simulink model "VL53L8A1_Full"  (R2024b)
settings: Solver=FixedStepDiscrete  StartTime=0.0  StopTime=inf  RelTol=1e-3  EnableMultiTasking=on
PreLoadFcn:
  | addpath(genpath(pwd))
InitFcn:
  | addpath(genpath(pwd));
  | auto_program("VL53L8A1_Full");
  | STLINK_COMPORT = auto_COMPORT()
  | 
  | dialogPrms = get_param(gcs+"/VL53L8A1", 'DialogParameters');
  | dialogPrmNames = fieldnames(dialogPrms);
  | odr4 = get_param(gcs+"/VL53L8A1", dialogPrmNames{1});
  | odr4 = eval(odr4);
  | 
  | STM32_ODR = odr4
  | clearvars -except STLINK_COMPORT STLINK_DRIVE STM32_ODR
libraries: instrumentseriallib x3, etargetslib x3
settings Model: SimulationMode=accelerator  PacingRate=0.100000  ExtModeTrigDuration=10  Creator=JesseJabezArendse  LastModifiedBy=JesseJabezArendse
settings OptimizationCC: ReuseModelBlockBuffer=off  PassReuseOutputArgsAs=Individual arguments  ZeroExternalMemoryAtStartup=off  ZeroInternalMemoryAtStartup=off  MaxStackSize=64  OptimizationLevel=level1  OptimizationCustomize=off  EfficientTunableParamExpr=on
settings DebuggingCC: ParameterPrecisionLossMsg=none  ParameterTunabilityLossMsg=error
settings HardwareCC: ProdBitPerPointer=32  ProdBitPerSizeT=32  ProdBitPerPtrDiffT=32  ProdLargestAtomicInteger=Long  ProdLargestAtomicFloat=Double  ProdWordSize=32  ProdLongLongMode=on  ProdHWDeviceType=ARM Compatible->ARM Cortex
settings ModelReferenceCC: EnableParallelModelReferenceBuilds=on
settings SFSimCC: SimCustomHeaderCode="#include \"Core\\Inc\\main.h\""  SimParseCustomCode=off  MATLABDynamicMemAlloc=off  SimHardwareAcceleration=native
settings SFSimCC: SimUserSources=|
  | Core\Src\main.c
  | Core\Src\IKS02A1_Simulink.c
settings SFSimCC: SimUserIncludeDirs=|
  | Core\Inc\
  | Core\Src\
settings RTWCC: Description=Embedded Coder  SystemTargetFile=ert.tlc  TemplateMakefile=ert_default_tmf  RTWUseSimCustomCode=on  CustomHeaderCode="#include \"Core\\Inc\\main.h\""  Toolchain=GNU Tools for ARM Embedded Processors  BuildConfiguration=Specify  GPUComputeCapability=3.5
settings RTWCC: CustomInclude=|
  | Core\Inc\
  | Core\Src\
settings RTWCC: CustomSource=|
  | Core\Src\main.c
  | Core\Src\IKS02A1_Simulink.c
settings CodeAppCC: ForceParamTrailComments=on  IgnoreCustomStorageClasses=off  OperatorAnnotations=on  SimulinkDataObjDesc=on  SFDataObjDesc=on  InsertBlockDesc=on
settings ERTTargetCC: CodeReplacementLibrary=ARM Cortex-M  SupportContinuousTime=on  ExtModeTransport=3  ExtModeStaticAlloc=on  ExtModeStaticAllocSize=2000  ExtModeMexFile=ext_xcp  ExtModeIntrfLevel=Level2 - Open  InlinedParameterPlacement=Hierarchical  ERTCustomFileTemplate=example_file_process.tlc  DynamicArrayContainerType=coder::array

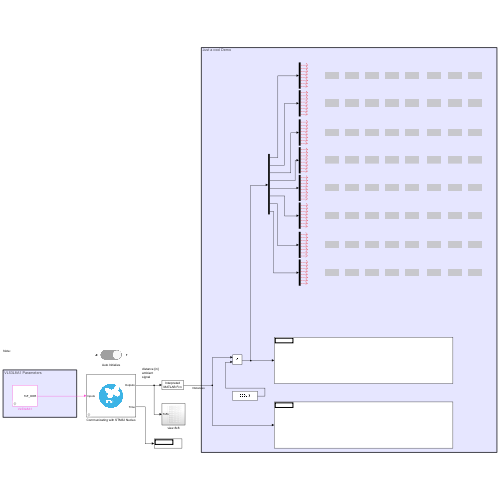
[thumbnail: Simulink's stored preview of the top-level diagram]
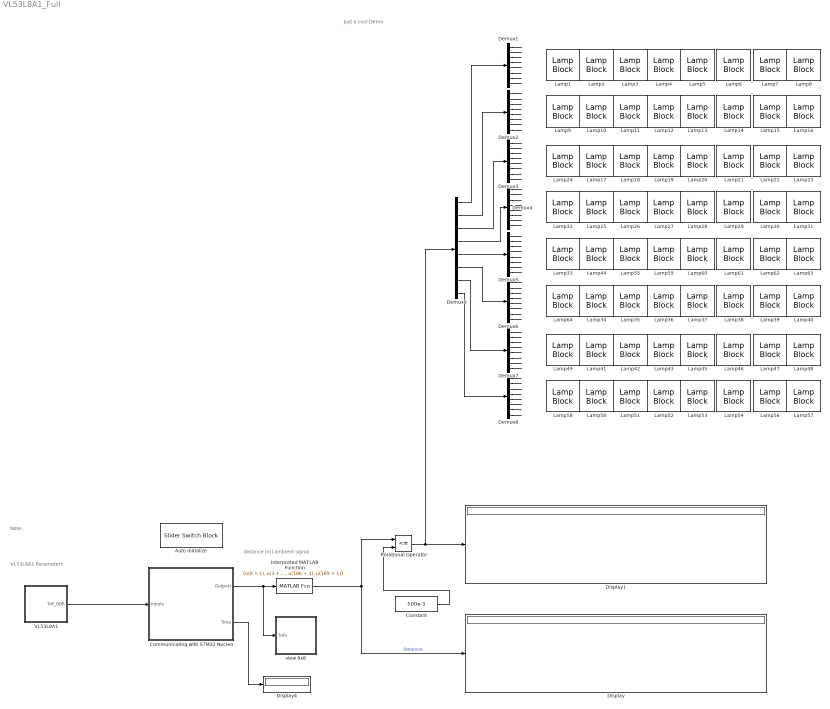
== system VL53L8A1_Full ==
  note: Just a cool Demo
  note: distance [m]
      | ambient
      | signal
  note: Note:
  note: VL53L8A1 Parameters
  Auto Initialize : SliderSwitchBlock  LabelPosition=Hide
      settings: Values={{'Off', 'On'}, [0 1]}
  Communicating with STM32 Nucleo : Subsystem  mask{Auto_Initialize=1}
      mask prompts: Auto_Initialize "Automate Initialization?"
      mask TypeOptions Auto_Initialize: 1 | 0
      mask DialogControl Control1 Prompt: Block for communication between host machine and STM32 Nucleo F411RE
      mask Display: image('stm32_icon.png', [0,0,0,0,80,80]);
  Constant : Constant  Value=500e-3
  Demux0 : Demux  Outputs=[8 8 8 8 8 8 8 8]
  Demux{1..8} (8 alike) : Demux  Outputs=[1 1 1 1 1 1 1 1]
  Display : Display
  Display1 : Display
  Display4 : Display
  Interpreted MATLAB Function : MATLABFcn  MATLABFcn=|
      | [u(0 + 1),
      | u(3 + 1),
      | u(6 + 1),
      | u(9 + 1),
      | u(12 + 1),
      | u(15 + 1),
      | u(18 + 1),
      | u(21 + 1),
      | u(24 + 1),
      | u(27 + 1),
      | u(30 + 1),
      | u(33 + 1),
      | u(36 + 1),
      | u(39 + 1),
      | u(42 + 1),
      | u(45 + 1),
      | u(48 + 1),
      | u(51 + 1),
      | u(54 + 1),
      | u(57 + 1),
      | u(60 + 1),
      | u(63 + 1),
      | u(66 + 1),
      | u(69 + 1),
      | u(72 + 1),
      | u(75 + 1),
      | u(78 + 1),
      | u(81 + 1),
      | u(84 + 1),
      | u(87 + 1),
      | u(90 + 1),
      | u(93 + 1),
      | u(96 + 1),
      | u(99 + 1),
      | u(102 + 1),
      | u(105 + 1),
      | u(108 + 1),
      | u(111 + 1),
      | u(114 + 1),
      | u(117 + 1),
      | u(120 + 1),
      | u(123 + 1),
      | u(126 + 1),
      | u(129 + 1),
      | u(132 + 1),
      | u(135 + 1),
      | u(138 + 1),
      | u(141 + 1),
      | u(144 + 1),
      | u(147 + 1),
      | u(150 + 1),
      | u(153 + 1),
      | u(156 + 1),
      | u(159 + 1),
      | u(162 + 1),
      | u(165 + 1),
      | u(168 + 1),
      | u(171 + 1),
      | u(174 + 1),
      | u(177 + 1),
      | u(180 + 1),
      | u(183 + 1),
      | u(186 + 1),
      | u(189 + 1)]
  Lamp{1..64} (64 alike) : LampBlock  LabelPosition=Hide  Icon=Rectangle
  Relational Operator : RelationalOperator  Operator=<=  OutDataTypeStr=boolean  RndMeth=Simplest  InputSameDT=off
  VL53L8A1 : Subsystem  mask{ODR_TOF=20}
      mask prompts: ODR_TOF "Output Data Rate (Hz)"
      mask DialogControl DescGroupVar Prompt: Time of Flight Sensor 8x8
  view 8x8 : Subsystem
  wires:
  Interpreted MATLAB Function/1 -> Relational Operator/1, Display/1  "Distances"
  Constant/1 -> Relational Operator/2
  Demux1/1 -> ?
  Demux1/2 -> ?
  Demux1/3 -> ?
  Demux1/4 -> ?
  Demux1/5 -> ?
  Demux1/6 -> ?
  Demux1/7 -> ?
  Demux1/8 -> ?
  Relational Operator/1 -> Display1/1, Demux0/1
  Demux0/1 -> Demux1/1
  Demux2/8 -> ?
  Demux2/7 -> ?
  Demux2/6 -> ?
  Demux2/5 -> ?
  Demux2/4 -> ?
  Demux2/3 -> ?
  Demux2/2 -> ?
  Demux2/1 -> ?
  Demux0/2 -> Demux2/1
  Demux3/1 -> ?
  Demux3/3 -> ?
  Demux3/6 -> ?
  Demux3/2 -> ?
  Demux3/4 -> ?
  Demux3/5 -> ?
  Demux3/8 -> ?
  Demux0/3 -> Demux3/1
  Demux3/7 -> ?
  Demux4/2 -> ?
  Demux4/6 -> ?
  Demux4/1 -> ?
  Demux4/8 -> ?
  Demux4/5 -> ?
  Demux4/3 -> ?
  Demux4/7 -> ?
  Demux4/4 -> ?
  Demux0/4 -> Demux4/1
  Demux6/1 -> ?
  Demux6/2 -> ?
  Demux6/7 -> ?
  Demux6/4 -> ?
  Demux6/8 -> ?
  Demux5/3 -> ?
  Demux5/5 -> ?
  Demux6/6 -> ?
  Demux5/6 -> ?
  Demux7/2 -> ?
  Demux7/6 -> ?
  Demux6/3 -> ?
  Demux7/1 -> ?
  Demux5/7 -> ?
  Demux6/5 -> ?
  Demux5/8 -> ?
  Demux7/5 -> ?
  Demux7/8 -> ?
  Demux8/4 -> ?
  Demux8/1 -> ?
  Demux8/8 -> ?
  Demux7/7 -> ?
  Demux7/4 -> ?
  Demux8/3 -> ?
  Demux5/4 -> ?
  Demux8/7 -> ?
  Demux8/6 -> ?
  Demux7/3 -> ?
  Demux8/5 -> ?
  Demux8/2 -> ?
  Demux5/1 -> ?
  Demux5/2 -> ?
  Demux0/5 -> Demux5/1
  Demux0/6 -> Demux6/1
  Demux0/7 -> Demux7/1
  Demux0/8 -> Demux8/1
  Communicating with STM32 Nucleo/2(Time) -> Display4/1
  Communicating with STM32 Nucleo/1(Outputs) -> view 8x8/1(ToFs), Interpreted MATLAB Function/1
  VL53L8A1/1(ToF_ODR) -> Communicating with STM32 Nucleo/1(Inputs)

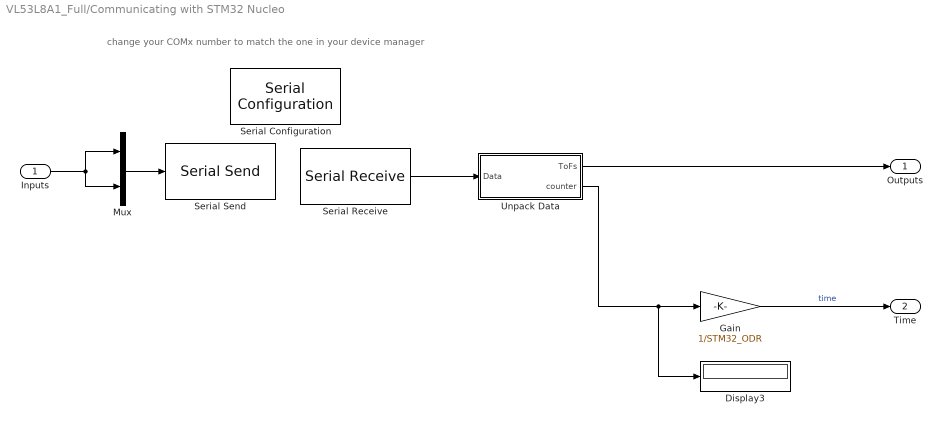
== system VL53L8A1_Full/Communicating with STM32 Nucleo ==
  note: change your COMx number to match the one in your device manager
  Inputs : Inport
  Display3 : Display
  Gain : Gain  Gain=1/STM32_ODR
  Mux : Mux  Inputs=2
  Serial Configuration : instrumentseriallib/Serial Configuration  Priority=-200000  PortSel=STLINK_COMPORT  Port=STLINK_COMPORT  ComPort=STLINK_COMPORT  BaudRate=1843200  DataBits=8  Parity=even  StopBits=2  ByteOrder=little-endian  FlowControl=none  Timeout=5  SimulateUsing=Interpreted execution  BlockInModel=on  aMode=1
      settings: LibrarySourceBlock=embeddedtargetslib/Host Communication/Serial Configuration
  Serial Receive : instrumentseriallib/Serial Receive  Priority=1  PortSel=STLINK_COMPORT  Port=STLINK_COMPORT  ComPort=STLINK_COMPORT  DataType=single  SaveDataType=uint8  ToggleHeader=on  Header='J_A'  ToggleDataSize=on  DataSize=[1 8*8*3+1]  ToggleTerminator=on  Terminator=Custom terminator  CustomTerminator='A_J'  InputFormat=Column major  EnableBlockingMode=on  ActionDataUnavailable=Output last received value  ActionWhenDataUnavailable=Output last received value  CustomValue=0  SampleTime=1/STM32_ODR  SimulateUsing=Interpreted execution  BlockInModel=on  aMode=1
      settings: LibrarySourceBlock=embeddedtargetslib/Host Communication/Serial Receive
  Serial Send : instrumentseriallib/Serial Send  Priority=1  PortSel=STLINK_COMPORT  Port=STLINK_COMPORT  ComPort=STLINK_COMPORT  Header='J_A'  Terminator=Custom terminator  CustomTerminator='A_J'  EnableBlockingMode=off  SimulateUsing=Interpreted execution  BlockInModel=on  aMode=1
      settings: LibrarySourceBlock=embeddedtargetslib/Host Communication/Serial Send
  Unpack Data : Subsystem
  Outputs : Outport
  Time : Outport  Port=2
  wires:
  Serial Receive/1 -> Unpack Data/1(Data)
  Gain/1 -> Time/1  "time"
  Inputs/1 -> Mux/1, Mux/2
  Unpack Data/1(ToFs) -> Outputs/1
  Unpack Data/2(counter) -> Gain/1, Display3/1
  Mux/1 -> Serial Send/1

== system VL53L8A1_Full/VL53L8A1 ==
  Byte Pack3 : etargetslib/Byte Pack  datatypes={'single'}  byteAlign=1
  Cast5 : DataTypeConversion  OutDataTypeStr=single  SaturateOnIntegerOverflow=off  RndMeth=Floor
  Constant1 : Constant  Value=ODR_TOF
  Display1 : Display
  ToF_ODR : Outport
  wires:
  Constant1/1 -> Cast5/1, Display1/1
  Cast5/1 -> Byte Pack3/1
  Byte Pack3/1 -> ToF_ODR/1

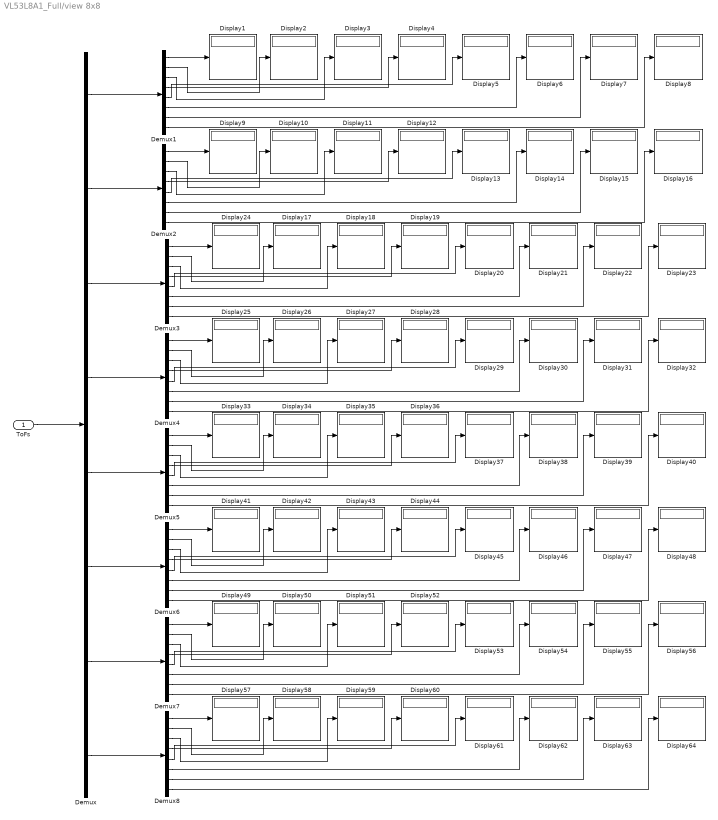
== system VL53L8A1_Full/view 8x8 ==
  ToFs : Inport
  Demux : Demux  Outputs=[3*8 3*8 3*8 3*8 3*8 3*8 3*8 3*8]
  Demux{1..8} (8 alike) : Demux  Outputs=[3 3 3 3 3 3 3 3]
  Display{1..64} (64 alike) : Display
  wires:
  Demux5/7 -> Display39/1
  Demux4/2 -> Display26/1
  Demux3/3 -> Display18/1
  Demux8/6 -> Display62/1
  Demux3/2 -> Display17/1
  Demux2/2 -> Display10/1
  Demux/5 -> Demux5/1
  Demux1/5 -> Display5/1
  Demux4/4 -> Display28/1
  Demux4/7 -> Display31/1
  Demux4/6 -> Display30/1
  Demux7/7 -> Display55/1
  Demux3/4 -> Display19/1
  Demux/8 -> Demux8/1
  Demux4/8 -> Display32/1
  Demux/4 -> Demux4/1
  Demux8/8 -> Display64/1
  Demux8/3 -> Display59/1
  Demux3/8 -> Display23/1
  Demux4/3 -> Display27/1
  Demux6/4 -> Display44/1
  Demux5/1 -> Display33/1
  Demux1/3 -> Display3/1
  Demux3/7 -> Display22/1
  Demux3/6 -> Display21/1
  Demux1/2 -> Display2/1
  Demux3/5 -> Display20/1
  Demux8/2 -> Display58/1
  Demux/1 -> Demux1/1
  Demux3/1 -> Display24/1
  Demux/2 -> Demux2/1
  Demux7/3 -> Display51/1
  Demux2/5 -> Display13/1
  Demux4/1 -> Display25/1
  Demux1/6 -> Display6/1
  Demux1/8 -> Display8/1
  Demux2/3 -> Display11/1
  Demux5/4 -> Display36/1
  Demux7/6 -> Display54/1
  Demux4/5 -> Display29/1
  Demux/6 -> Demux6/1
  Demux/3 -> Demux3/1
  Demux7/5 -> Display53/1
  Demux5/8 -> Display40/1
  Demux8/7 -> Display63/1
  Demux6/7 -> Display47/1
  Demux5/2 -> Display34/1
  Demux1/7 -> Display7/1
  Demux8/4 -> Display60/1
  Demux6/1 -> Display41/1
  Demux5/5 -> Display37/1
  Demux6/3 -> Display43/1
  Demux6/6 -> Display46/1
  Demux6/2 -> Display42/1
  Demux6/5 -> Display45/1
  Demux1/1 -> Display1/1
  Demux6/8 -> Display48/1
  Demux1/4 -> Display4/1
  Demux8/1 -> Display57/1
  Demux5/6 -> Display38/1
  Demux8/5 -> Display61/1
  Demux5/3 -> Display35/1
  Demux2/8 -> Display16/1
  Demux7/4 -> Display52/1
  Demux7/8 -> Display56/1
  Demux7/1 -> Display49/1
  Demux7/2 -> Display50/1
  Demux2/7 -> Display15/1
  Demux2/6 -> Display14/1
  Demux2/1 -> Display9/1
  Demux2/4 -> Display12/1
  Demux/7 -> Demux7/1
  ToFs/1 -> Demux/1

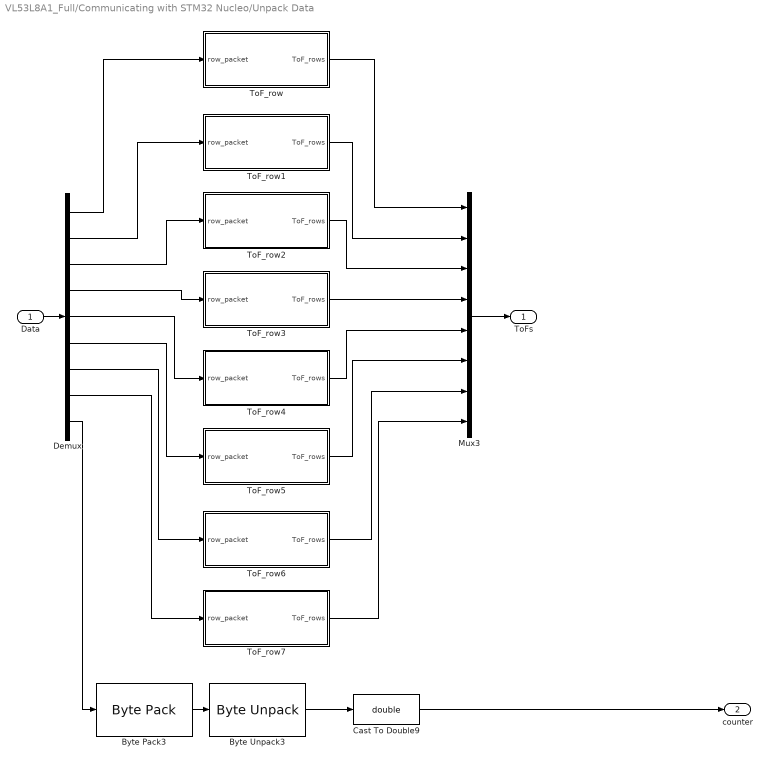
== system VL53L8A1_Full/Communicating with STM32 Nucleo/Unpack Data ==
  Data : Inport
  Byte Pack3 : etargetslib/Byte Pack  datatypes={'single'}  byteAlign=1
  Byte Unpack3 : etargetslib/Byte Unpack  dimensions={[1]}  datatypes={'uint32'}  byteAlign=1
      settings: LibrarySourceBlock=embeddedtargetslib/Host Communication/Byte Unpack
  Cast To Double9 : DataTypeConversion  OutDataTypeStr=double  SaturateOnIntegerOverflow=off  RndMeth=Floor
  Demux : Demux  Outputs=[3*8 3*8 3*8 3*8 3*8 3*8 3*8 3*8 1]
  Mux3 : Mux  Inputs=[3*8 3*8 3*8 3*8 3*8 3*8 3*8 3*8]
  ToF_row : Subsystem
  ToF_row1 : Subsystem
  ToF_row2 : Subsystem
  ToF_row3 : Subsystem
  ToF_row4 : Subsystem
  ToF_row5 : Subsystem
  ToF_row6 : Subsystem
  ToF_row7 : Subsystem
  ToFs : Outport
  counter : Outport  Port=2
  wires:
  Data/1 -> Demux/1
  Demux/7 -> ToF_row6/1(row_packet)
  Demux/6 -> ToF_row5/1(row_packet)
  Demux/5 -> ToF_row4/1(row_packet)
  Mux3/1 -> ToFs/1
  Demux/4 -> ToF_row3/1(row_packet)
  Demux/3 -> ToF_row2/1(row_packet)
  Demux/2 -> ToF_row1/1(row_packet)
  Demux/1 -> ToF_row/1(row_packet)
  Demux/8 -> ToF_row7/1(row_packet)
  ToF_row/1(ToF_rows) -> Mux3/1
  ToF_row1/1(ToF_rows) -> Mux3/2
  ToF_row2/1(ToF_rows) -> Mux3/3
  ToF_row3/1(ToF_rows) -> Mux3/4
  ToF_row4/1(ToF_rows) -> Mux3/5
  ToF_row5/1(ToF_rows) -> Mux3/6
  ToF_row6/1(ToF_rows) -> Mux3/7
  ToF_row7/1(ToF_rows) -> Mux3/8
  Demux/9 -> Byte Pack3/1
  Byte Unpack3/1 -> Cast To Double9/1
  Cast To Double9/1 -> counter/1
  Byte Pack3/1 -> Byte Unpack3/1

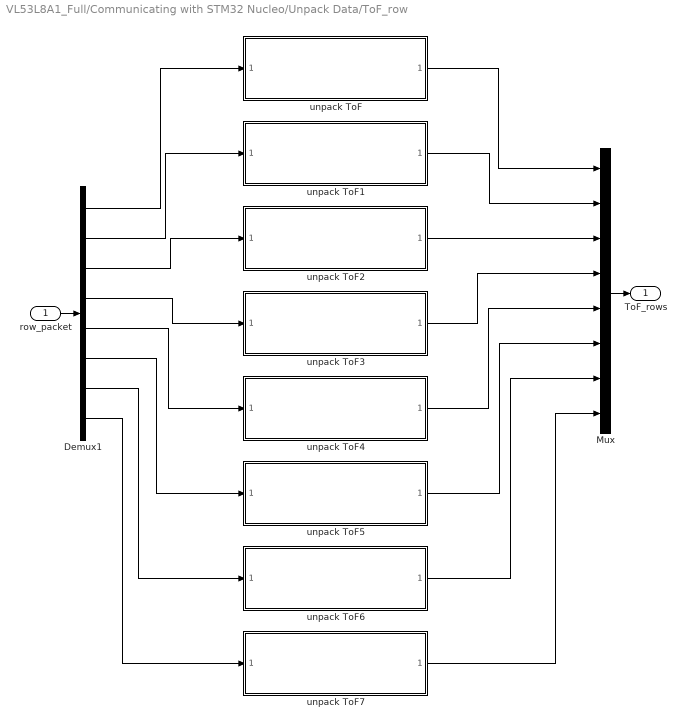
== system VL53L8A1_Full/Communicating with STM32 Nucleo/Unpack Data/ToF_row ==
  row_packet : Inport
  Demux1 : Demux  Outputs=[3 3 3 3 3 3 3 3]
  Mux : Mux  Inputs=[3 3 3 3 3 3 3 3]
  unpack ToF{,1..7} (8 alike) : Subsystem  ReferencedSubsystem=unpack_ToF
  ToF_rows : Outport
  wires:
  Demux1/7 -> unpack ToF6/1
  unpack ToF5/1 -> Mux/6
  unpack ToF3/1 -> Mux/4
  Demux1/1 -> unpack ToF/1
  Demux1/8 -> unpack ToF7/1
  Demux1/3 -> unpack ToF2/1
  Demux1/5 -> unpack ToF4/1
  Demux1/2 -> unpack ToF1/1
  unpack ToF1/1 -> Mux/2
  Demux1/4 -> unpack ToF3/1
  unpack ToF4/1 -> Mux/5
  unpack ToF7/1 -> Mux/8
  Mux/1 -> ToF_rows/1
  Demux1/6 -> unpack ToF5/1
  unpack ToF6/1 -> Mux/7
  unpack ToF/1 -> Mux/1
  unpack ToF2/1 -> Mux/3
  row_packet/1 -> Demux1/1

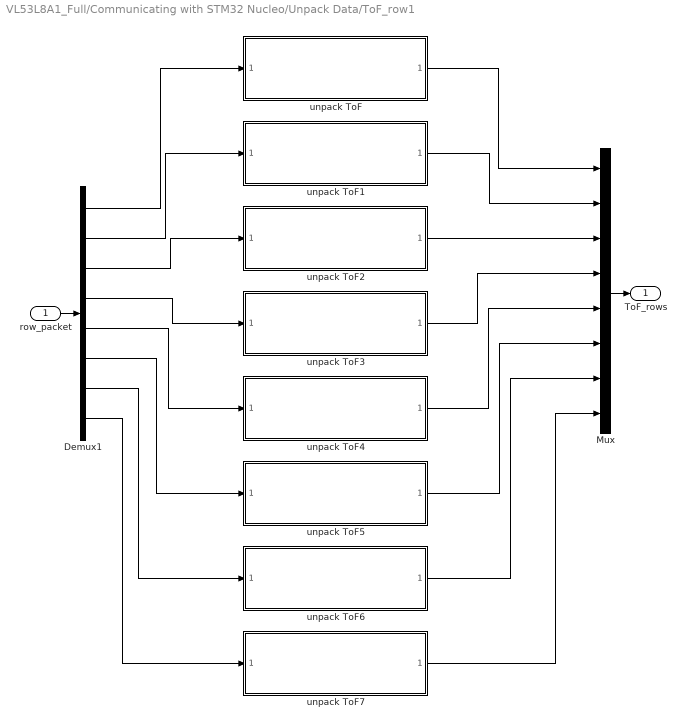
== system VL53L8A1_Full/Communicating with STM32 Nucleo/Unpack Data/ToF_row1 ==
  row_packet : Inport
  Demux1 : Demux  Outputs=[3 3 3 3 3 3 3 3]
  Mux : Mux  Inputs=[3 3 3 3 3 3 3 3]
  unpack ToF{,1..7} (8 alike) : Subsystem  ReferencedSubsystem=unpack_ToF
  ToF_rows : Outport
  wires:
  row_packet/1 -> Demux1/1
  unpack ToF2/1 -> Mux/3
  unpack ToF/1 -> Mux/1
  unpack ToF6/1 -> Mux/7
  Demux1/6 -> unpack ToF5/1
  Mux/1 -> ToF_rows/1
  unpack ToF7/1 -> Mux/8
  unpack ToF4/1 -> Mux/5
  Demux1/4 -> unpack ToF3/1
  unpack ToF1/1 -> Mux/2
  Demux1/2 -> unpack ToF1/1
  Demux1/5 -> unpack ToF4/1
  Demux1/3 -> unpack ToF2/1
  Demux1/8 -> unpack ToF7/1
  Demux1/1 -> unpack ToF/1
  unpack ToF3/1 -> Mux/4
  unpack ToF5/1 -> Mux/6
  Demux1/7 -> unpack ToF6/1

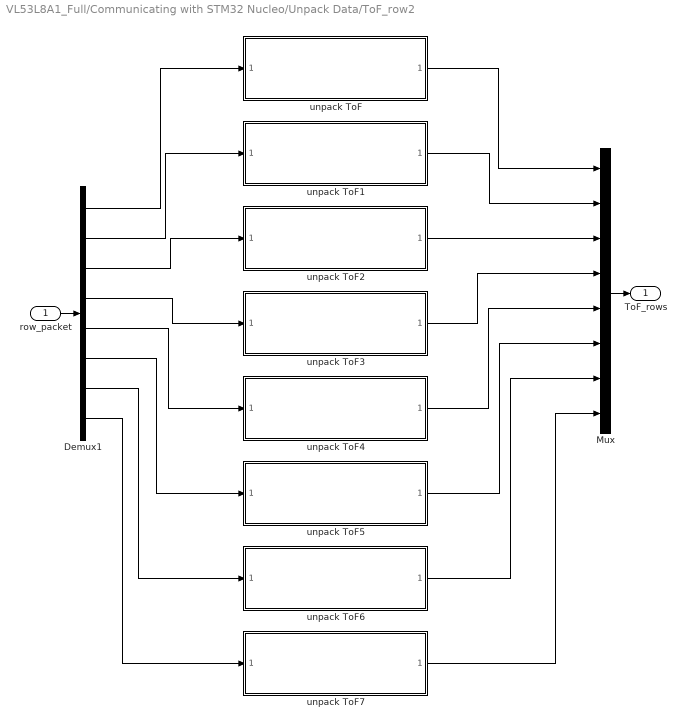
== system VL53L8A1_Full/Communicating with STM32 Nucleo/Unpack Data/ToF_row2 ==
  row_packet : Inport
  Demux1 : Demux  Outputs=[3 3 3 3 3 3 3 3]
  Mux : Mux  Inputs=[3 3 3 3 3 3 3 3]
  unpack ToF{,1..7} (8 alike) : Subsystem  ReferencedSubsystem=unpack_ToF
  ToF_rows : Outport
  wires:
  Demux1/7 -> unpack ToF6/1
  unpack ToF5/1 -> Mux/6
  unpack ToF3/1 -> Mux/4
  Demux1/1 -> unpack ToF/1
  Demux1/8 -> unpack ToF7/1
  Demux1/3 -> unpack ToF2/1
  Demux1/5 -> unpack ToF4/1
  Demux1/2 -> unpack ToF1/1
  unpack ToF1/1 -> Mux/2
  Demux1/4 -> unpack ToF3/1
  unpack ToF4/1 -> Mux/5
  unpack ToF7/1 -> Mux/8
  Mux/1 -> ToF_rows/1
  Demux1/6 -> unpack ToF5/1
  unpack ToF6/1 -> Mux/7
  unpack ToF/1 -> Mux/1
  unpack ToF2/1 -> Mux/3
  row_packet/1 -> Demux1/1

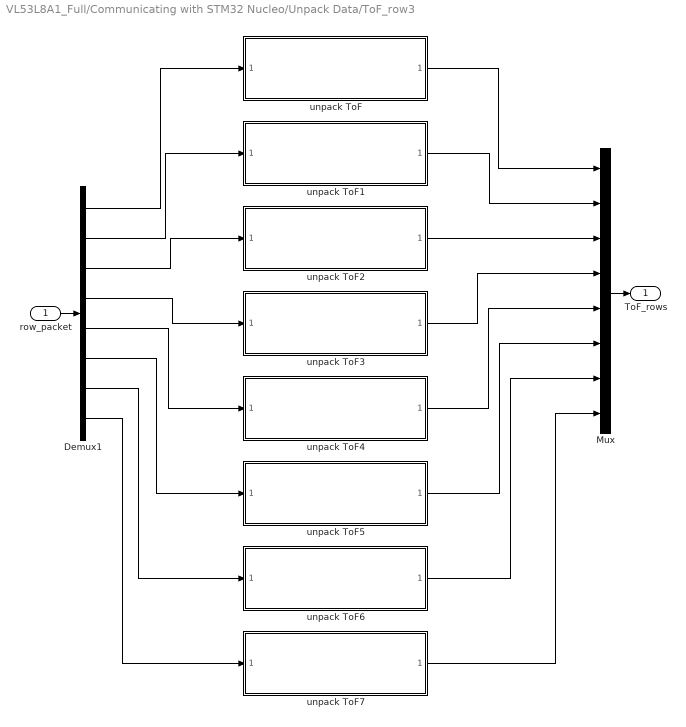
== system VL53L8A1_Full/Communicating with STM32 Nucleo/Unpack Data/ToF_row3 ==
  row_packet : Inport
  Demux1 : Demux  Outputs=[3 3 3 3 3 3 3 3]
  Mux : Mux  Inputs=[3 3 3 3 3 3 3 3]
  unpack ToF{,1..7} (8 alike) : Subsystem  ReferencedSubsystem=unpack_ToF
  ToF_rows : Outport
  wires:
  row_packet/1 -> Demux1/1
  unpack ToF2/1 -> Mux/3
  unpack ToF/1 -> Mux/1
  unpack ToF6/1 -> Mux/7
  Demux1/6 -> unpack ToF5/1
  Mux/1 -> ToF_rows/1
  unpack ToF7/1 -> Mux/8
  unpack ToF4/1 -> Mux/5
  Demux1/4 -> unpack ToF3/1
  unpack ToF1/1 -> Mux/2
  Demux1/2 -> unpack ToF1/1
  Demux1/5 -> unpack ToF4/1
  Demux1/3 -> unpack ToF2/1
  Demux1/8 -> unpack ToF7/1
  Demux1/1 -> unpack ToF/1
  unpack ToF3/1 -> Mux/4
  unpack ToF5/1 -> Mux/6
  Demux1/7 -> unpack ToF6/1

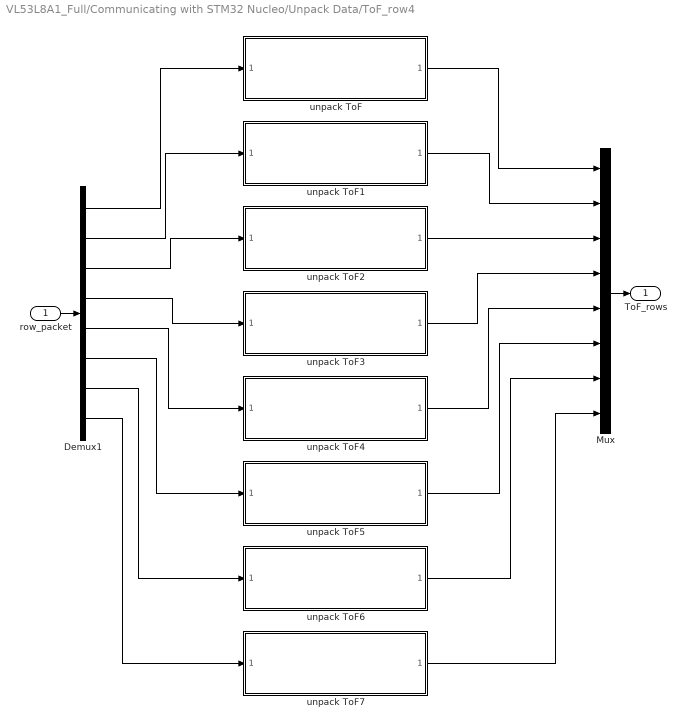
== system VL53L8A1_Full/Communicating with STM32 Nucleo/Unpack Data/ToF_row4 ==
  row_packet : Inport
  Demux1 : Demux  Outputs=[3 3 3 3 3 3 3 3]
  Mux : Mux  Inputs=[3 3 3 3 3 3 3 3]
  unpack ToF{,1..7} (8 alike) : Subsystem  ReferencedSubsystem=unpack_ToF
  ToF_rows : Outport
  wires:
  Demux1/7 -> unpack ToF6/1
  unpack ToF5/1 -> Mux/6
  unpack ToF3/1 -> Mux/4
  Demux1/1 -> unpack ToF/1
  Demux1/8 -> unpack ToF7/1
  Demux1/3 -> unpack ToF2/1
  Demux1/5 -> unpack ToF4/1
  Demux1/2 -> unpack ToF1/1
  unpack ToF1/1 -> Mux/2
  Demux1/4 -> unpack ToF3/1
  unpack ToF4/1 -> Mux/5
  unpack ToF7/1 -> Mux/8
  Mux/1 -> ToF_rows/1
  Demux1/6 -> unpack ToF5/1
  unpack ToF6/1 -> Mux/7
  unpack ToF/1 -> Mux/1
  unpack ToF2/1 -> Mux/3
  row_packet/1 -> Demux1/1

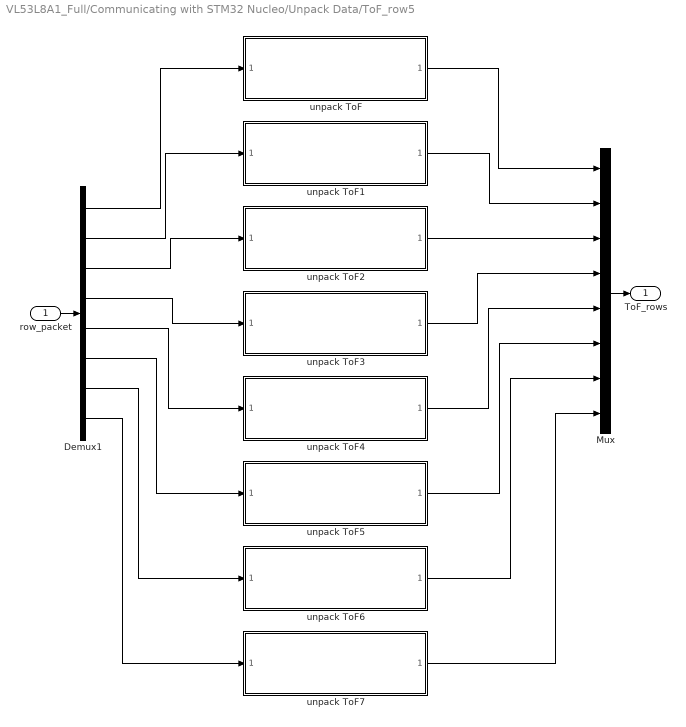
== system VL53L8A1_Full/Communicating with STM32 Nucleo/Unpack Data/ToF_row5 ==
  row_packet : Inport
  Demux1 : Demux  Outputs=[3 3 3 3 3 3 3 3]
  Mux : Mux  Inputs=[3 3 3 3 3 3 3 3]
  unpack ToF{,1..7} (8 alike) : Subsystem  ReferencedSubsystem=unpack_ToF
  ToF_rows : Outport
  wires:
  row_packet/1 -> Demux1/1
  unpack ToF2/1 -> Mux/3
  unpack ToF/1 -> Mux/1
  unpack ToF6/1 -> Mux/7
  Demux1/6 -> unpack ToF5/1
  Mux/1 -> ToF_rows/1
  unpack ToF7/1 -> Mux/8
  unpack ToF4/1 -> Mux/5
  Demux1/4 -> unpack ToF3/1
  unpack ToF1/1 -> Mux/2
  Demux1/2 -> unpack ToF1/1
  Demux1/5 -> unpack ToF4/1
  Demux1/3 -> unpack ToF2/1
  Demux1/8 -> unpack ToF7/1
  Demux1/1 -> unpack ToF/1
  unpack ToF3/1 -> Mux/4
  unpack ToF5/1 -> Mux/6
  Demux1/7 -> unpack ToF6/1

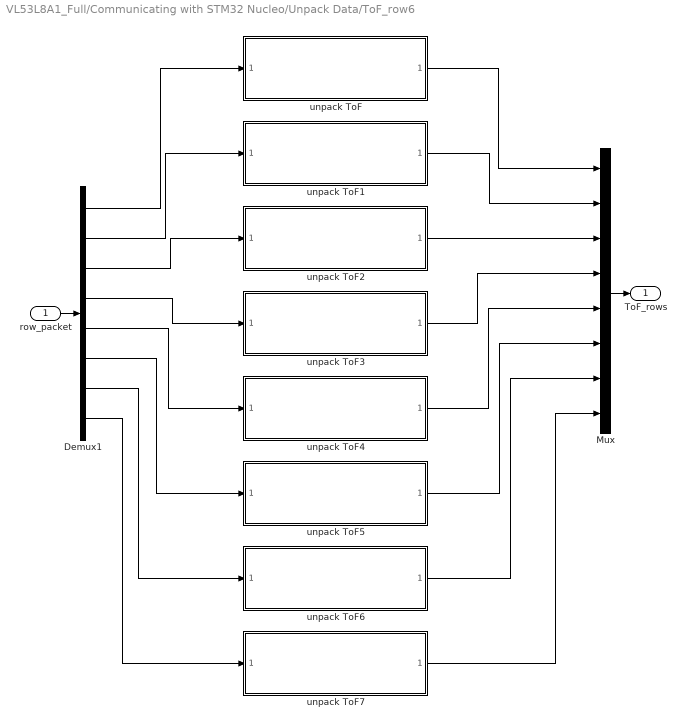
== system VL53L8A1_Full/Communicating with STM32 Nucleo/Unpack Data/ToF_row6 ==
  row_packet : Inport
  Demux1 : Demux  Outputs=[3 3 3 3 3 3 3 3]
  Mux : Mux  Inputs=[3 3 3 3 3 3 3 3]
  unpack ToF{,1..7} (8 alike) : Subsystem  ReferencedSubsystem=unpack_ToF
  ToF_rows : Outport
  wires:
  Demux1/7 -> unpack ToF6/1
  unpack ToF5/1 -> Mux/6
  unpack ToF3/1 -> Mux/4
  Demux1/1 -> unpack ToF/1
  Demux1/8 -> unpack ToF7/1
  Demux1/3 -> unpack ToF2/1
  Demux1/5 -> unpack ToF4/1
  Demux1/2 -> unpack ToF1/1
  unpack ToF1/1 -> Mux/2
  Demux1/4 -> unpack ToF3/1
  unpack ToF4/1 -> Mux/5
  unpack ToF7/1 -> Mux/8
  Mux/1 -> ToF_rows/1
  Demux1/6 -> unpack ToF5/1
  unpack ToF6/1 -> Mux/7
  unpack ToF/1 -> Mux/1
  unpack ToF2/1 -> Mux/3
  row_packet/1 -> Demux1/1

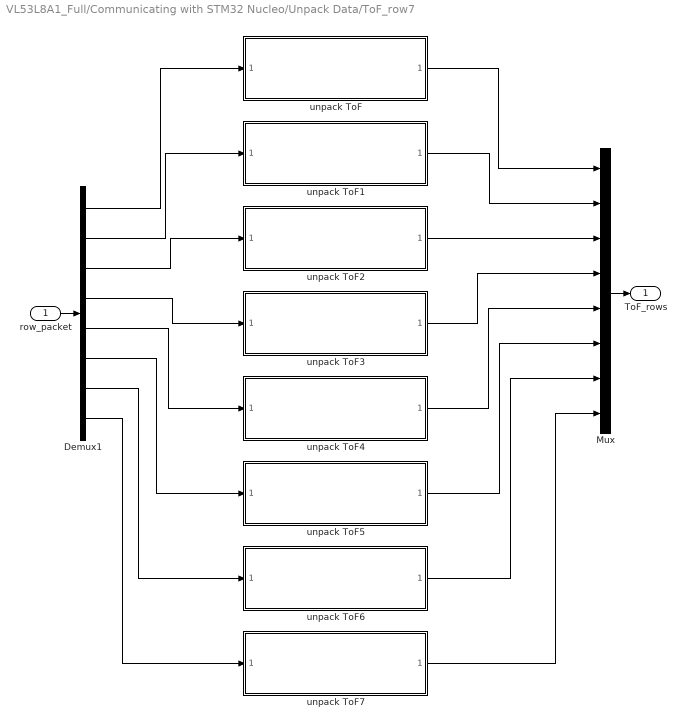
== system VL53L8A1_Full/Communicating with STM32 Nucleo/Unpack Data/ToF_row7 ==
  row_packet : Inport
  Demux1 : Demux  Outputs=[3 3 3 3 3 3 3 3]
  Mux : Mux  Inputs=[3 3 3 3 3 3 3 3]
  unpack ToF{,1..7} (8 alike) : Subsystem  ReferencedSubsystem=unpack_ToF
  ToF_rows : Outport
  wires:
  row_packet/1 -> Demux1/1
  unpack ToF2/1 -> Mux/3
  unpack ToF/1 -> Mux/1
  unpack ToF6/1 -> Mux/7
  Demux1/6 -> unpack ToF5/1
  Mux/1 -> ToF_rows/1
  unpack ToF7/1 -> Mux/8
  unpack ToF4/1 -> Mux/5
  Demux1/4 -> unpack ToF3/1
  unpack ToF1/1 -> Mux/2
  Demux1/2 -> unpack ToF1/1
  Demux1/5 -> unpack ToF4/1
  Demux1/3 -> unpack ToF2/1
  Demux1/8 -> unpack ToF7/1
  Demux1/1 -> unpack ToF/1
  unpack ToF3/1 -> Mux/4
  unpack ToF5/1 -> Mux/6
  Demux1/7 -> unpack ToF6/1
